simulink model "LQG"  (R2017b)
settings: Solver=FixedStepAuto  StartTime=0.0  StopTime=10.0  FixedStep=0.01  RelTol=1e-3
values from neighbouring files (symbols this model uses):
  A = [0 1 0 0 ... (first row only)    [Untitled.m]
  B = [0;-1/M;0;1/M]    [Untitled.m]
  C = [1 0 0 0;0 0 1 0]    [Untitled.m]
  K = lqr(A,B,Q,R)    [Untitled.m]
  L = lqe(A,G,C,Qn, Rn)    [Untitled.m]
libraries: simulink x2
settings Model: Creator=DELL  LastModifiedBy=DELL

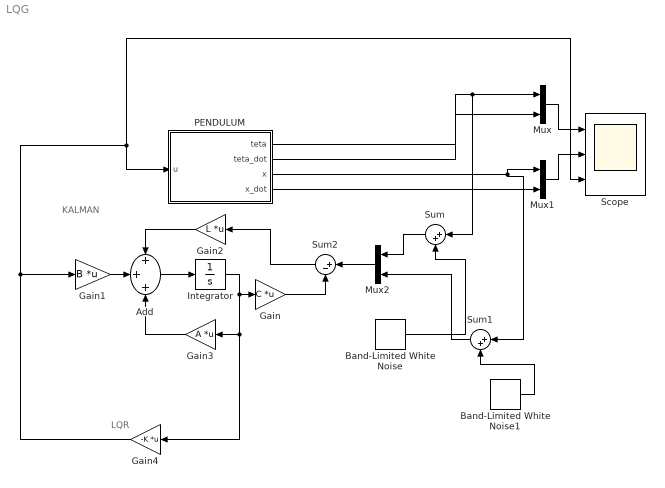
== system LQG ==
  note: KALMAN
  note: LQR
  Add : Sum  Inputs=+++
  Band-Limited White Noise : simulink/Sources/Band-Limited White Noise  Cov=[0.00001]  Ts=0.01  seed=[23341]
  Band-Limited White Noise1 : simulink/Sources/Band-Limited White Noise  Cov=[0.01]  Ts=0.01  seed=[23341]
  Gain : Gain  Gain=C  Multiplication=Matrix(K*u)
  Gain1 : Gain  Gain=B  Multiplication=Matrix(K*u)
  Gain2 : Gain  Gain=L  Multiplication=Matrix(K*u)
  Gain3 : Gain  Gain=A  Multiplication=Matrix(K*u)
  Gain4 : Gain  Gain=-K  Multiplication=Matrix(K*u)
  Integrator : Integrator
  Mux : Mux  Inputs=2
  Mux1 : Mux  Inputs=2
  Mux2 : Mux  Inputs=2
  PENDULUM : Subsystem
  Scope : Scope  NumInputPorts=3
  Sum : Sum  Inputs=|++
  Sum1 : Sum  Inputs=|++
  Sum2 : Sum  Inputs=|+-
  wires:
  Mux/1 -> Scope/1
  Mux1/1 -> Scope/2
  PENDULUM/1(teta) -> Sum/1, Mux/1
  PENDULUM/2(teta_dot) -> Mux/2
  PENDULUM/3(x) -> Mux1/1, Sum1/1
  PENDULUM/4(x_dot) -> Mux1/2
  Band-Limited White Noise/1 -> Sum/2
  Band-Limited White Noise1/1 -> Sum1/2
  Sum/1 -> Mux2/1
  Sum1/1 -> Mux2/2
  Mux2/1 -> Sum2/1
  Add/1 -> Integrator/1
  Integrator/1 -> Gain4/1, Gain3/1, Gain/1
  Gain/1 -> Sum2/2
  Sum2/1 -> Gain2/1
  Gain2/1 -> Add/1
  Gain3/1 -> Add/3
  Gain1/1 -> Add/2
  Gain4/1 -> PENDULUM/1(u), Scope/3, Gain1/1

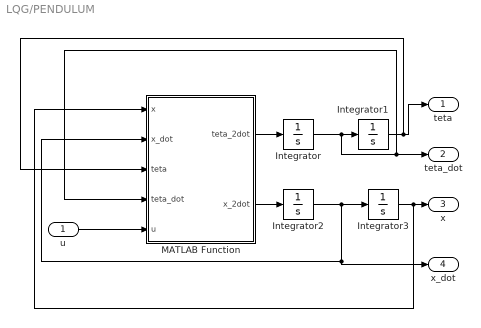
== system LQG/PENDULUM ==
  u : Inport
  Integrator : Integrator
  Integrator1 : Integrator  InitialCondition=0.2
  Integrator2 : Integrator
  Integrator3 : Integrator
  MATLAB Function : MATLAB Function  TreatAsAtomicUnit=on
  teta : Outport
  teta_dot : Outport  Port=2
  x : Outport  Port=3
  x_dot : Outport  Port=4
  wires:
  u/1 -> MATLAB Function/5(u)
  MATLAB Function/2(x_2dot) -> Integrator2/1
  Integrator2/1 -> MATLAB Function/2(x_dot), x_dot/1, Integrator3/1
  MATLAB Function/1(teta_2dot) -> Integrator/1
  Integrator/1 -> teta_dot/1, MATLAB Function/4(teta_dot), Integrator1/1
  Integrator1/1 -> MATLAB Function/3(teta), teta/1
  Integrator3/1 -> MATLAB Function/1(x), x/1

== matlab function LQG/PENDULUM/MATLAB Function ==
  data: x input; x_dot input; teta input; teta_dot input; u input; teta_2dot output; x_2dot output
%Program by Tran Van The HCMUTE 
% 5/11/2023
function [teta_2dot,x_2dot] = Pendulum(x,x_dot,teta,teta_dot,u)
M = 1;
m = 0.1;
g = 9.81;
l = 1;


x_2dot=(u+m*l*sin(teta)*(teta_dot)^2-m*g*sin(teta)*cos(teta))/(M+m-m*cos(teta)^2);
teta_2dot=(u*cos(teta)-(M+m)*g*sin(teta)+m*l*(sin(teta)*cos(teta))*(teta_dot)^2)/(m*l*cos(teta)^2-(M+m)*l);
